simulink model "FrequencyComparator_Rx"  (R2020a)
settings: Solver=FixedStepDiscrete  StartTime=0.0  StopTime=inf  RelTol=1e-3  EnableMultiTasking=on
undefined symbols (not defined in the file): Fs, ip, usb
libraries: plutoradiolib x1, dspspect3 x1
settings Model: DataTypeOverride=Off  Creator=The MathWorks, Inc.  LastModifiedBy=juanj
settings SolverCC: PositivePriorityOrder=on  AutoInsertRateTranBlk=on
settings DataIOCC: LimitDataPoints=on  SaveFormat=Array  ReturnWorkspaceOutputs=off
settings OptimizationCC: UseDivisionForNetSlopeComputation=on  GainParamInheritBuiltInType=on  UseFloatMulNetSlope=on  EnhancedBackFolding=on  PassReuseOutputArgsAs=Individual arguments  ExpressionDepthLimit=2147483647  ZeroExternalMemoryAtStartup=off  ZeroInternalMemoryAtStartup=off  EfficientFloat2IntCast=on  MaxStackSize=64  OptimizeBlockOrder=speed  DifferentSizesBufferReuse=on  OptimizationCustomize=off  EfficientTunableParamExpr=on
settings DebuggingCC: AlgebraicLoopMsg=error  UnderspecifiedInitializationDetection=Classic  MergeDetectMultiDrivingBlocksExec=none  SolverPrmCheckMsg=warning  SingleTaskRateTransMsg=error  ParameterPrecisionLossMsg=none  ParameterTunabilityLossMsg=error  FcnCallInpInsideContextMsg=warning  AllowSymbolicDim=off  StateNameClashWarn=warning  SFUnexpectedBacktrackingDiag=warning  SFNoUnconditionalDefaultTransitionDiag=warning  SFExecutionAtInitializationDiag=none  ArithmeticOperatorsInVariantConditions=warning
settings HardwareCC: ProdBitPerPointer=32  ProdBitPerSizeT=32  ProdBitPerPtrDiffT=32  ProdLargestAtomicInteger=Long  ProdLargestAtomicFloat=Double  ProdWordSize=32  ProdLongLongMode=on  ProdHWDeviceType=ARM Compatible->ARM Cortex  TargetBitPerPointer=64  TargetBitPerSizeT=64  TargetBitPerPtrDiffT=64  TargetLongLongMode=on  TargetIntDivRoundTo=Zero  TargetEndianess=LittleEndian  TargetWordSize=64  TargetHWDeviceType=Custom Processor->MATLAB Host Computer  ProdEqTarget=off
settings ModelReferenceCC: PropagateSignalLabelsOutOfModel=off
settings SFSimCC: SimUseLocalCustomCode=off  MATLABDynamicMemAlloc=off  CustomCodeUndefinedFunction=UseInterfaceOnly
settings RTWCC: SystemTargetFile=ert.tlc  HardwareBoard=ZedBoard  TemplateMakefile=ert_default_tmf  RTWUseLocalCustomCode=off  Toolchain=Linaro AArch32 Linux v6.3.1  BuildConfiguration=Faster Runs
settings RTWCC: CustomSourceCode=|
  | #include<stdio.h>
  | #include<stdlib.h>
settings CodeAppCC: ForceParamTrailComments=on  IgnoreCustomStorageClasses=off  OperatorAnnotations=on  SimulinkDataObjDesc=on  SFDataObjDesc=on  InsertBlockDesc=on
settings ConfigComp: CovMetricSettings=dw  CovHtmlReporting=on  CovSaveCumulativeToWorkspaceVar=on  CovSaveSingleToWorkspaceVar=on  CovExternalEMLEnable=off  CovSFcnEnable=off

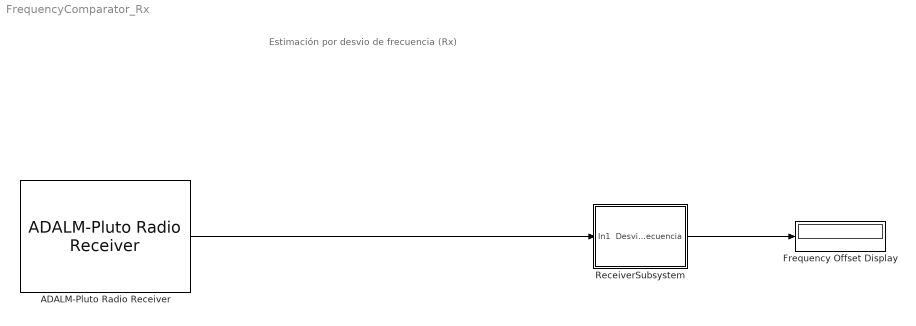
== system FrequencyComparator_Rx ==
  note: Estimación por desvio de frecuencia
      | (Rx)
  ADALM-Pluto Radio Receiver : plutoradiolib/ADALM-Pluto Radio Receiver  RadioID=usb:0  uri=ip:10.0.0.200  CenterFrequencySource=Dialog  CenterFrequency=900000740  GainSource=AGC Fast Attack  GainSourceBlock=AGC Slow Attack  Gain=20  ChannelMapping=1  BasebandSampleRate=100e3  OutputDataType=double  SamplesPerFrame=10000  OverflowOutputPort=off  EnableBurstMode=off  NumFramesInBurst=1  ShowAdvancedProperties=off  UseCustomFilter=off  filtPathRates=[737280000 11520000 3840000 1920000 960000 240000]  filtCoefficients=[-192 82 85 -215 228 -102 -110 290 -318 145 160 -426 471 -215 -238 633 -697 318 349 -923 1009 -457 -498 1309 -1423 640 693 -1812 1959 -876 -945 2458 -2647 1180 1268 -3290 3534 -1572 -1688 4375 -4698 2091 2247 -5836 6284 -2807 -3031 7918 -8588 3870 4225 -11182 12324 -5662 -6330 17255 -19735 9507 11312 -33568 43355 -25227 -42139 305542 305542 -42139 -25227 43355 -33568 11312 9507 -19735 17255 -6330 -5662 12324 -11182 4225 3870 -8588 7918 -3031 -2807 6284 -5836 2247 2091 -4698 4375 -1688 -1572 3534 -3290 1268 1180 -2647 2458 -945 -876 1959 -1812 693 640 -1423 1309 -498 -457 1009 -923 349 318 -697 633 -238 -215 471 -426 160 145 -318 290 -110 -102 228 -215 85 82 -192]  filtCoefficientSize=128  filtDecimInterpFactor=4  filtGain=-12  filtRFBandwidth=18000000  filterConfigStruct=struct()  EnableQuadratureCorrection=on  EnableRFDCCorrection=on  EnableBasebandDCCorrection=on  FrequencyCorrection=0  OverrideSampleTime=off  SampleTime=0.02  DataTimeout=Inf  ENSMPinControlMode=None  BISTLoopbackMode=Disabled  BISTToneInject=Disabled  BISTSignalGen=PRBS  BISTToneFreq=Fs/32  BISTToneLevel=0
      settings: SourceProductBaseCode=PLUTO
  Frequency Offset Display : Display
  ReceiverSubsystem : Subsystem
  wires:
  ReceiverSubsystem/1(Desvio de frecuencia) -> Frequency Offset Display/1
  ADALM-Pluto Radio Receiver/1 -> ReceiverSubsystem/1(In1)

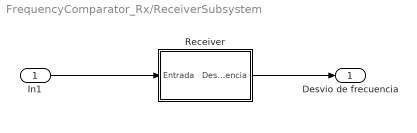
== system FrequencyComparator_Rx/ReceiverSubsystem ==
  In1 : Inport
  Receiver : Subsystem  TreatAsAtomicUnit=on
      mask Display: disp('Receiver')
  Desvio de frecuencia : Outport
  wires:
  In1/1 -> Receiver/1(Entrada)
  Receiver/1(Desvio de frecuencia) -> Desvio de frecuencia/1

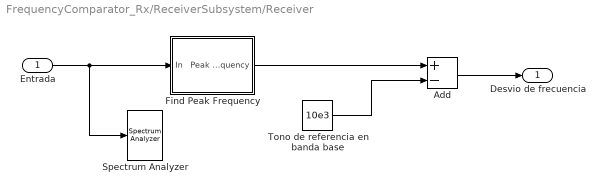
== system FrequencyComparator_Rx/ReceiverSubsystem/Receiver ==
  Entrada : Inport
  Add : Sum  Inputs=+-
  Find Peak Frequency : Subsystem
      mask Display: disp('Find Peak\nFrequency')
  Spectrum Analyzer : SpectrumAnalyzer
  Tono de referencia en banda base : Constant  Value=10e3
  Desvio de frecuencia : Outport  VectorParamsAs1DForOutWhenUnconnected=off
  wires:
  Find Peak Frequency/1(Peak Frequency) -> Add/1
  Tono de referencia en banda base/1 -> Add/2
  Add/1 -> Desvio de frecuencia/1
  Entrada/1 -> Spectrum Analyzer/1, Find Peak Frequency/1(In)

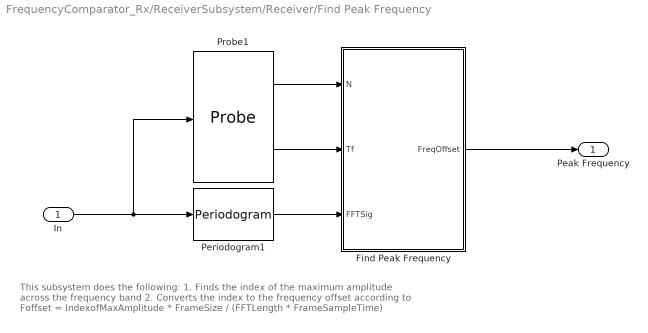
== system FrequencyComparator_Rx/ReceiverSubsystem/Receiver/Find Peak Frequency ==
  note: This subsystem does the following:
      | 1.  Finds the index of the maximum amplitude across the frequency band
      | 2.  Converts the index to the frequency offset according to
      | Foffset = IndexofMaxAmplitude * FrameSize / (FFTLength * FrameSampleTime)
  In : Inport
  Find Peak Frequency : MATLAB Function  TreatAsAtomicUnit=on
  Periodogram1 : dspspect3/Periodogram  measurement=Power spectral density  wintype=Hamming  Rs=50  beta=5  winsamp=Symmetric  FFTImplementation=Auto  inheritFFT=off  fftsize=2048  navg=2  inheritTs=on  Ts=1
      settings: SourceProductBaseCode=DS
  Probe1 : Probe  ProbeComplexSignal=off
  Peak Frequency : Outport  VectorParamsAs1DForOutWhenUnconnected=off
  wires:
  Periodogram1/1 -> Find Peak Frequency/3(FFTSig)
  Probe1/1 -> Find Peak Frequency/1(N)
  Probe1/2 -> Find Peak Frequency/2(Tf)
  Find Peak Frequency/1(FreqOffset) -> Peak Frequency/1
  In/1 -> Periodogram1/1, Probe1/1

== matlab function FrequencyComparator_Rx/ReceiverSubsystem/Receiver/Find Peak Frequency/Find Peak Frequency ==
  settings: fimath=fimath('RoundingMethod', 'Floor','OverflowAction', 'Wrap','ProductMode', 'FullPrecision', 'SumMode', 'FullPrecision')
  data: N input; FreqOffset output; Tf input; FFTSig input
function FreqOffset  = findpeakfreq(N, Tf, FFTSig)
% Find peak frequency
% N - frame size
% Tf - frame sample time
% FFTSig - result of FFT

%#codegen

FFTSize = length(FFTSig);
FFTSig = fftshift(FFTSig);
[~, maxIdx] = max(FFTSig); % Find index of max magnitude
OffsetIdx = maxIdx-1-FFTSize/2; % Convert to index symmetric with 0
Ts = Tf(1)/N; % Sample time
delta_f = 1/Ts/FFTSize; % Frequency resolution of FFT
FreqOffset = OffsetIdx*delta_f;% Map offset index back to frequency
